simulink model "nonlinear_Modell_21"  (R2021b)
settings: Solver=VariableStepAuto  StartTime=0.0  StopTime=20  RelTol=1e-3
values from neighbouring files (symbols this model uses):
  A = []    [equilibrium.m]
  u_eq1 = double(u_eq1)    [linearModel.m]
  x_eq = [1 15 70]    [linearModel.m]
undefined symbols (not defined in the file or in its folder): B, C, uss
libraries: slctrlblks x6
settings Model: Creator=derri  LastModifiedBy=sheng
settings DebuggingCC: UnconnectedInputMsg=none  UnconnectedOutputMsg=none  UnconnectedLineMsg=none
settings ModelReferenceCC: EnableRefExpFcnMdlSchedulingChecks=off
settings RTWCC: DLArmComputeVersion=20.02.1

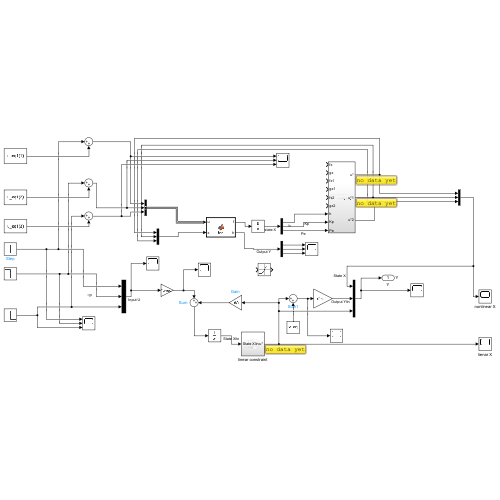
[thumbnail: Simulink's stored preview of the top-level diagram]
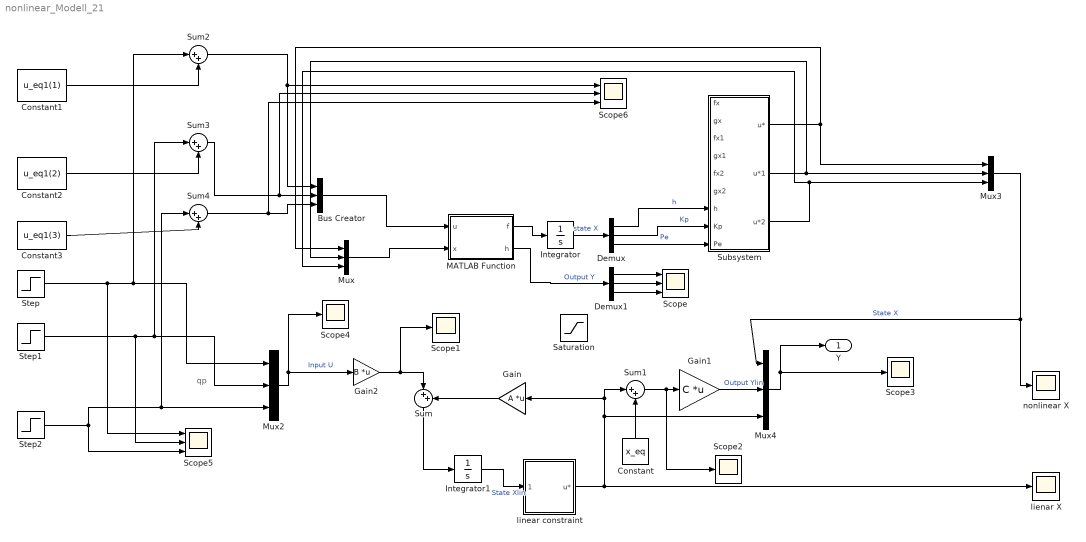
== system nonlinear_Modell_21 ==
  note: qp
  Bus Creator : BusCreator  Inputs=3
  Constant : Constant  Value=x_eq
  Constant1 : Constant  Value=u_eq1(1)
  Constant2 : Constant  Value=u_eq1(2)
  Constant3 : Constant  Value=u_eq1(3)
  Demux : Demux  Outputs=3
  Demux1 : Demux  Outputs=3
  Gain : Gain  Gain=A  Multiplication=Matrix(K*u)
  Gain1 : Gain  Gain=C  Multiplication=Matrix(K*u)
  Gain2 : Gain  Gain=B  Multiplication=Matrix(K*u) (u vector)
  Integrator : Integrator  InitialCondition=x_eq'
  Integrator1 : Integrator
  MATLAB Function : MATLAB Function  TreatAsAtomicUnit=on
  Mux{,2..4} (4 alike) : Mux  Inputs=3
  Saturation : Saturate
  Scope : Scope  NumInputPorts=3
  Scope{1..4} (4 alike) : Scope
  Scope5 : Scope  NumInputPorts=3
  Scope6 : Scope  NumInputPorts=3
  Step : Step  Time=0  After=uss(1)  SampleTime=0
  Step1 : Step  Time=0  After=uss(2)  SampleTime=0
  Step2 : Step  Time=0  After=uss(3)  SampleTime=0
  Subsystem : Subsystem
  Sum{,1..4} (5 alike) : Sum  Inputs=|++
  lienar X : Scope
  linear constraint : Subsystem
  nonlinear X : Scope
  Y : Outport  SignalName=Y
  wires:
  Demux/1 -> Subsystem/7(h)  "h"
  Demux/2 -> Subsystem/8(Kp)  "Kp"
  Demux/3 -> Subsystem/9(Pe)  "Pe"
  Mux/1 -> MATLAB Function/2(x)
  Demux1/1 -> Scope/1
  Demux1/2 -> Scope/2
  Demux1/3 -> Scope/3
  MATLAB Function/2(h) -> Demux1/1  "Output Y"
  MATLAB Function/1(f) -> Integrator/1
  Sum/1 -> Integrator1/1
  Gain1/1 -> Mux4/2  "Output Ylin"
  Mux3/1 -> Mux4/1, nonlinear X/1  "State X"
  Mux4/1 -> Y/1, Scope3/1
  Integrator/1 -> Demux/1  "state X"
  Gain2/1 -> Scope1/1, Sum/1
  Constant/1 -> Sum1/2
  Mux2/1 -> Gain2/1, Scope4/1  "Input U"
  Sum1/1 -> Gain1/1, Scope2/1
  Gain/1 -> Sum/2
  Step/1 -> Sum2/1, Mux2/1, Scope5/1
  Step1/1 -> Sum3/1, Mux2/2, Scope5/2
  Step2/1 -> Mux2/3, Sum4/1, Scope5/3
  Constant1/1 -> Sum2/2
  Bus Creator/1 -> MATLAB Function/1(u)
  Sum2/1 -> Bus Creator/1, Scope6/1
  Sum3/1 -> Scope6/2, Bus Creator/2
  Sum4/1 -> Bus Creator/3, Scope6/3
  Constant2/1 -> Sum3/2
  Constant3/1 -> Sum4/2
  Subsystem/1(u*) -> Mux/1, Mux3/1
  Subsystem/2(u*1) -> Mux3/2, Mux/2
  Subsystem/3(u*2) -> Mux/3, Mux3/3
  linear constraint/1(u*) -> lienar X/1, Mux4/3, Gain/1, Sum1/1
  Integrator1/1 -> linear constraint/1(State Xlin)  "State Xlin"

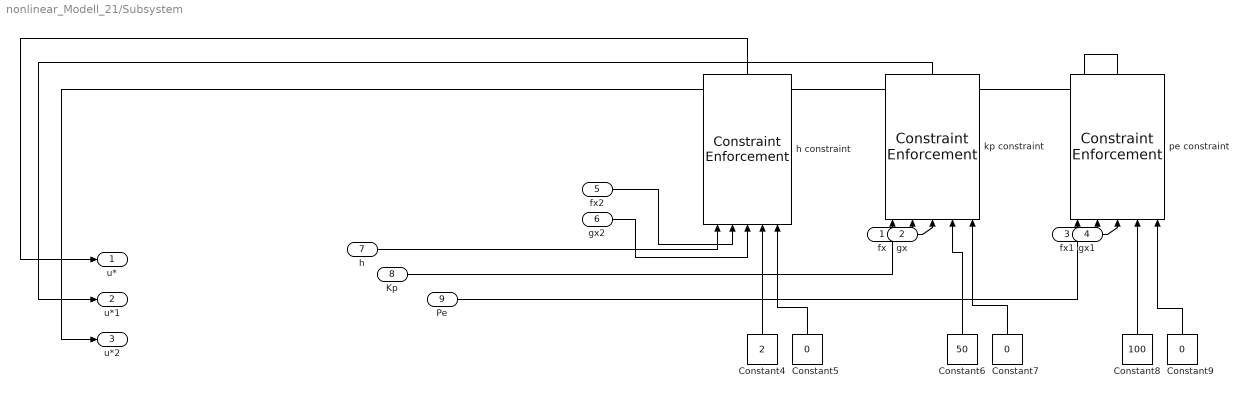
== system nonlinear_Modell_21/Subsystem ==
  fx : Inport
  gx : Inport  Port=2
  fx1 : Inport  Port=3
  gx1 : Inport  Port=4
  fx2 : Inport  Port=5
  gx2 : Inport  Port=6
  h : Inport  Port=7
  Kp : Inport  Port=8
  Pe : Inport  Port=9
  Constant4 : Constant  Value=2
  Constant5 : Constant  Value=0
  Constant6 : Constant  Value=50
  Constant7 : Constant  Value=0
  Constant8 : Constant  Value=100
  Constant9 : Constant  Value=0
  h constraint : slctrlblks/Constraint Enforcement  nc=1  nu=1  c=0  external_c=off  external_umax=on  external_umin=on  Ts=0.1  maxiter=200  tol=1e-6  output_exitflag=off  relax_c=off  relax_u=off
      settings: SourceProductBaseCode=SD
  kp constraint : slctrlblks/Constraint Enforcement  nc=1  nu=1  c=0  external_c=off  external_umax=on  external_umin=on  Ts=0.1  maxiter=200  tol=1e-6  output_exitflag=off  relax_c=off  relax_u=off
      settings: SourceProductBaseCode=SD
  pe constraint : slctrlblks/Constraint Enforcement  nc=1  nu=1  c=0  external_c=off  external_umax=on  external_umin=on  Ts=0.1  maxiter=200  tol=1e-6  output_exitflag=off  relax_c=off  relax_u=off
      settings: SourceProductBaseCode=SD
  u* : Outport
  u*1 : Outport  Port=2
  u*2 : Outport  Port=3
  wires:
  Constant6/1 -> kp constraint/4
  pe constraint/1 -> u*2/1
  Constant5/1 -> h constraint/5
  h/1 -> h constraint/1
  fx2/1 -> h constraint/2
  Constant9/1 -> pe constraint/5
  Kp/1 -> kp constraint/1
  Constant4/1 -> h constraint/4
  Constant8/1 -> pe constraint/4
  Constant7/1 -> kp constraint/5
  h constraint/1 -> u*/1
  Pe/1 -> pe constraint/1
  fx/1 -> kp constraint/2
  kp constraint/1 -> u*1/1
  fx1/1 -> pe constraint/2
  gx1/1 -> pe constraint/3
  gx/1 -> kp constraint/3
  gx2/1 -> h constraint/3

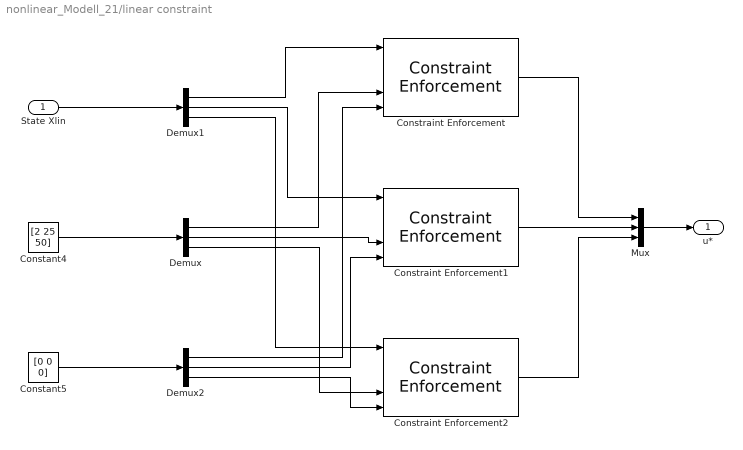
== system nonlinear_Modell_21/linear constraint ==
  State Xlin : Inport
  Constant4 : Constant  Value=[2 25 50]
  Constant5 : Constant  Value=[0 0 0]
  Constraint Enforcement : slctrlblks/Constraint Enforcement  nc=1  nu=1  c=0  external_c=off  external_umax=on  external_umin=on  Ts=0.1  maxiter=200  tol=1e-6  output_exitflag=off  relax_c=off  relax_u=off
      settings: SourceProductBaseCode=SD
  Constraint Enforcement1 : slctrlblks/Constraint Enforcement  nc=1  nu=1  c=0  external_c=off  external_umax=on  external_umin=on  Ts=0.1  maxiter=200  tol=1e-6  output_exitflag=off  relax_c=off  relax_u=off
      settings: SourceProductBaseCode=SD
  Constraint Enforcement2 : slctrlblks/Constraint Enforcement  nc=1  nu=1  c=0  external_c=off  external_umax=on  external_umin=on  Ts=0.1  maxiter=200  tol=1e-6  output_exitflag=off  relax_c=off  relax_u=off
      settings: SourceProductBaseCode=SD
  Demux : Demux  Outputs=3
  Demux1 : Demux  Outputs=3
  Demux2 : Demux  Outputs=3
  Mux : Mux  Inputs=3
  u* : Outport
  wires:
  Constant4/1 -> Demux/1
  State Xlin/1 -> Demux1/1
  Constant5/1 -> Demux2/1
  Demux1/1 -> Constraint Enforcement/1
  Demux1/2 -> Constraint Enforcement1/1
  Demux1/3 -> Constraint Enforcement2/1
  Demux/1 -> Constraint Enforcement/4
  Demux/2 -> Constraint Enforcement1/4
  Demux/3 -> Constraint Enforcement2/4
  Demux2/1 -> Constraint Enforcement/5
  Demux2/2 -> Constraint Enforcement1/5
  Demux2/3 -> Constraint Enforcement2/5
  Constraint Enforcement1/1 -> Mux/2
  Mux/1 -> u*/1
  Constraint Enforcement/1 -> Mux/1
  Constraint Enforcement2/1 -> Mux/3

== matlab function nonlinear_Modell_21/MATLAB Function ==
  data: f output; h output; u input; x input
function [f,h] = fcn(u,x)
p=getparam_Gsp();
u1=u(1);
u2=u(2);
u3=u(3);
x1=x(1);
x2=x(2);
x3=x(3);
f=[p.a1*x3+p.a2*x2-p.b1*u1-p.b2*(u2+p.K*x1)-p.k1;...
-p.a3*x2*(u2+p.K*x1)+p.k2;...
-p.a4*x3-p.a5*x2+p.b3*u1-((p.a6*x3+p.b4)/(p.b5*u3+p.k3))*u3+p.k4
];
h=[x1; x2; x3];
